simulink model "LQRSimulink"  (R2025b)
settings: Solver=VariableStepAuto  StartTime=0.0  StopTime=30  RelTol=1e-3
values from neighbouring files (symbols this model uses):
  K = dcgain(G_quadrata)    [estrai_tfm.m]
undefined symbols (not defined in the file or in its folder): A_long, B_long
libraries: aerolibfltsims x2
settings Model: Creator=leonardoleggeri  LastModifiedBy=leonardoleggeri

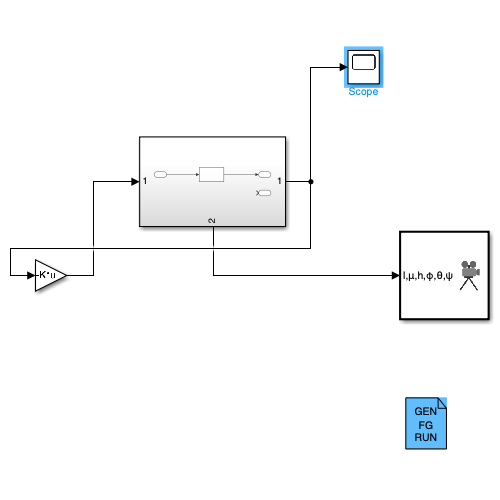
[thumbnail: Simulink's stored preview of the top-level diagram]
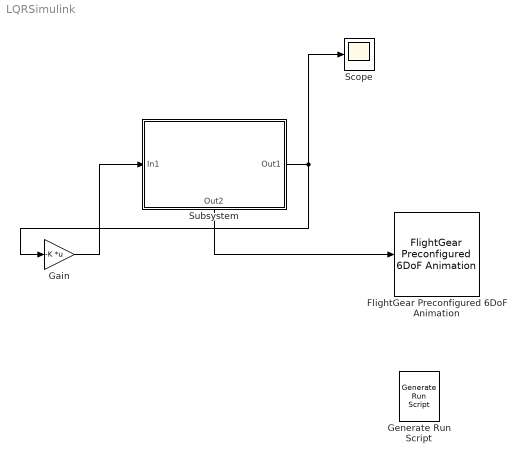
== system LQRSimulink ==
  FlightGear Preconfigured 6DoF Animation : aerolibfltsims/FlightGear Preconfigured 6DoF Animation  xFlightGearVersion=v2019.1  DestinationIpAddress=127.0.0.1  DestinationPort=5502  SampleTime=1/30  packetVersion=24
  Gain : Gain  Gain=-K  Multiplication=Matrix(K*u)
  Generate Run Script : aerolibfltsims/Generate Run Script  Architecture=Default  dataFlow=Send  GeometryModelName=HL20  AirportId=KSFO  RunwayId=10L  InitialAltitude=7224  InitialHeading=113  OffsetDistance=4.72  OffsetAzimuth=0  InstallScenery=off  DisableShaders=off  OriginAddress=127.0.0.1  DestinationPort=5502  OriginPort=5505  LocalAddress=127.0.0.1  OutputFileName=runfg.bat  FlightGearBaseDirectory=C:\Program Files\FlightGear
  Scope : Scope
      settings: ActiveDisplayYMinimum=-3.9001884517964678  ActiveDisplayYMaximum=9.264325290734865
  Subsystem : Subsystem
      settings: PortSchema="{\"entries\":[{\"content\":{\"sides\":[{\"content\":{\"connectorIds\":[\"In1\"]},\"type\":\"ConnectorPlacement.EquallySpacedRectSide\",\"uuid\":\"5543c79e-e828-4d10-8402-177b2277ecee\"},{\"content\":{\"connectorIds\":[\"Out1\"],\"side\":\"RIGHT\"},\"type\":\"ConnectorPlacement.EquallySpacedRectSide\",\"uuid\":\"edfc78c0-967f-4077-8890-f746e92e6a35\"},{\"content\":{\"side\":\"TOP\"},\"type\":\"ConnectorPlacement.EquallySpacedRectSide\",\"uuid\":\"9ff6976c-09b7-430e-96e3-20e6ab76c101\"},{\"content\":{\"connectorIds\":[\"Out2\"],\"side\":\"BOTTOM\"},\"type\":\"ConnectorPlacement.EquallySpacedRectSide\",\"uuid\":\"e341721d-1b86-47bc-9f00-b8897cbbd2c1\"}]},\"type\":\"ConnectorPlacement.EquallySpacedConnector\",\"uuid\":\"703acde8-523c-4d05-8f32-d89cf934eef3\"}],\"packageUris\":[\"http://schema.mathworks.com/mf0/Connector/R2020b\"],\"version\":\"1.0\"}"
  wires:
  Subsystem/1(Out1) -> Gain/1, Scope/1
  Gain/1 -> Subsystem/1(In1)
  Subsystem/2(Out2) -> FlightGear Preconfigured 6DoF Animation/1

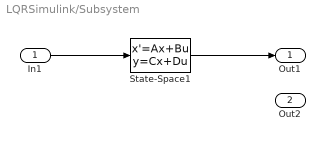
== system LQRSimulink/Subsystem ==
  In1 : Inport
  State-Space1 : StateSpace  A=A_long  B=B_long  C=eye(4)  D=zeros(4,5)  InitialCondition=[0.4; 0.2; 30; 15]
  Out1 : Outport
  Out2 : Outport  Port=2
  wires:
  In1/1 -> State-Space1/1
  State-Space1/1 -> Out1/1
